simulink model "FKtest"  (Simulink 6.6)
settings: Solver=ode4  StartTime=0.0  StopTime=400  FixedStep=0.05  RelTol=1e-3
undefined symbols (not defined in the file or in its folder): amp2, vessel
libraries: marine_gnc x21, simulink x5
(part 2 of 3)

== system FKtest/Subsystem2/Subsystem ==
  In1 : Inport
  In2 : Inport  Port=2
  Integrator : Integrator
  Product4 : Product  Inputs=*/  RndMeth=Zero
  Out1 : Outport
  wires:
  Integrator/1 -> Product4/1
  In1/1 -> Integrator/1
  Product4/1 -> Out1/1
  In2/1 -> Product4/2

== system FKtest/Subsystem2/Subsystem1 ==
  In1 : Inport
  In2 : Inport  Port=2
  Integrator : Integrator
  Product4 : Product  Inputs=*/  RndMeth=Zero
  Out1 : Outport
  wires:
  Integrator/1 -> Product4/1
  In1/1 -> Integrator/1
  Product4/1 -> Out1/1
  In2/1 -> Product4/2

== system FKtest/Subsystem3/Subsystem ==
  In1 : Inport
  In2 : Inport  Port=2
  Integrator : Integrator
  Product4 : Product  Inputs=*/  RndMeth=Zero
  Out1 : Outport
  wires:
  Integrator/1 -> Product4/1
  In1/1 -> Integrator/1
  Product4/1 -> Out1/1
  In2/1 -> Product4/2

== system FKtest/Subsystem3/Subsystem1 ==
  In1 : Inport
  In2 : Inport  Port=2
  Integrator : Integrator
  Product4 : Product  Inputs=*/  RndMeth=Zero
  Out1 : Outport
  wires:
  Integrator/1 -> Product4/1
  In1/1 -> Integrator/1
  Product4/1 -> Out1/1
  In2/1 -> Product4/2

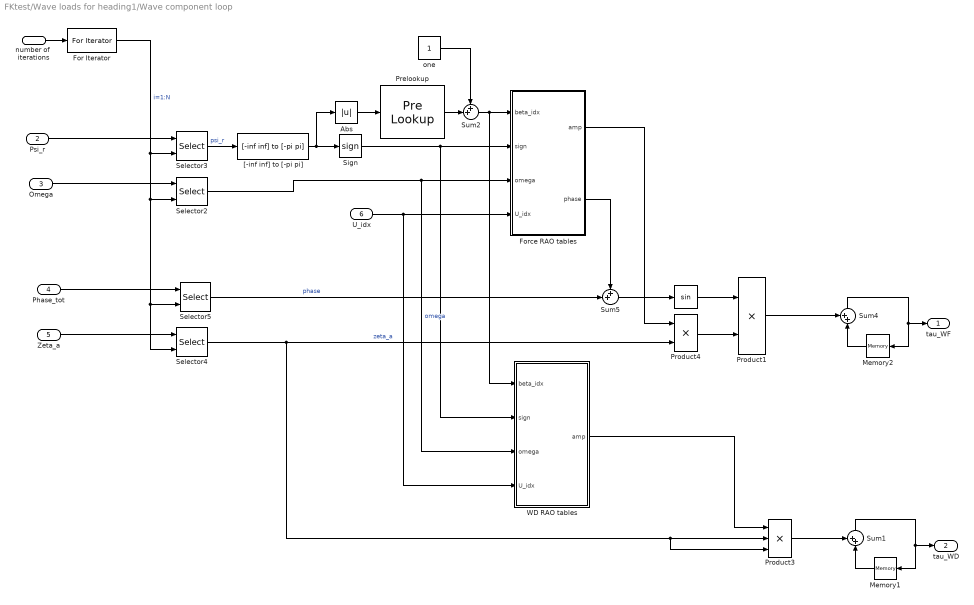
== system FKtest/Wave loads for heading1/Wave component loop ==
  number of  iterations : Inport
  Psi_r : Inport  Port=2
  Omega : Inport  Port=3
  Phase_tot : Inport  Port=4
  Zeta_a : Inport  Port=5
  U_idx : Inport  Port=6
  "                " : Trigonometry
  Abs : Abs  SaturateOnIntegerOverflow=on
  For Iterator : ForIterator  ResetStates=reset  IterationSource=external  IterationVariableDataType=double
  Force RAO tables : Subsystem  AncestorBlock=marine_gnc/Models/Environmental Loads/Utilities/RAO tables  mask(RAO table lookup){RAO_Freq=ForceRAO_Freq, RAO_Dir=RAO_Dir, RAO_Vel=RAO_Vel, RAO_Amp=ForceRAO_Amp, RAO_Phase=ForceRAO_Phase}
      mask prompts: RAO_Freq "Vector of frequencies (rad/s)"; RAO_Dir "Vector of directions (rad)"; RAO_Vel "Vector of velocities (m/s)"; RAO_Amp "6DOF Cell array with tables of Amplitudes"; RAO_Phase "6DOF Cell array with tables of Phases (rad)"
      mask help:
      | Perform 3D table lookup in 6DOF RAO amplitudes and phases, using the relative wave heading psi_r, wave frequency omega and vessel velocity vel as inputs. See documentation of the Motion RAO block or Force RAO block for details. A warning is issued if the input is outside the range spanned by the RAOs.
      |
      | Copyright (C) NTNU 2005
      |
      | Author: Oyvind N. Smogeli, 2005-05-03
  Memory1 : Memory  Orientation=left  X0=[0 0 0 0 0 0]'  InheritSampleTime=on
  Memory2 : Memory  Orientation=left  X0=[0 0 0 0 0 0]'  InheritSampleTime=on
  Prelookup : PreLookup  BreakpointsData=vessel.headings  BeginIndexSearchUsingPreviousIndexResult=on  OutputOnlyTheIndex=on
  Product1 : Product  SaturateOnIntegerOverflow=on
  Product3 : Product  Inputs=3  SaturateOnIntegerOverflow=on
  Product4 : Product  SaturateOnIntegerOverflow=on
  Selector{2..5} (4 alike) : Selector  IndexOptions=Index vector (port)  Indices=[1 3]  OutputSizes=1
  Sign : Signum
  Sum1 : Sum  Orientation=up  Inputs=++|  SaturateOnIntegerOverflow=on
  Sum2 : Sum  Inputs=++|
  Sum4 : Sum  Orientation=up  Inputs=++|  SaturateOnIntegerOverflow=on
  Sum5 : Sum  Inputs=++|  SaturateOnIntegerOverflow=on
  WD RAO tables : Subsystem  AncestorBlock=marine_gnc/Models/Environmental Loads/Utilities/RAO tables  mask(RAO table lookup){RAO_Freq=ForceRAO_Freq, RAO_Dir=RAO_Dir, RAO_Vel=RAO_Vel, RAO_Amp=ForceRAO_Amp, RAO_Phase=ForceRAO_Phase}
      mask prompts: RAO_Freq "Vector of frequencies (rad/s)"; RAO_Dir "Vector of directions (rad)"; RAO_Vel "Vector of velocities (m/s)"; RAO_Amp "6DOF Cell array with tables of Amplitudes"; RAO_Phase "6DOF Cell array with tables of Phases (rad)"
      mask help:
      | Perform 3D table lookup in 6DOF RAO amplitudes and phases, using the relative wave heading psi_r, wave frequency omega and vessel velocity vel as inputs. See documentation of the Motion RAO block or Force RAO block for details. A warning is issued if the input is outside the range spanned by the RAOs.
      |
      | Copyright (C) NTNU 2005
      |
      | Author: Oyvind N. Smogeli, 2005-05-03
  "[-inf inf] to [-pi pi]" : marine_gnc/Utilities/Math Operations/[-inf inf] to [-pi pi]  SystemSampleTime=-1
  one : Constant
  tau_WF : Outport
  tau_WD : Outport  Port=2
  wires:
  Selector4/1 -> Product4/2, Product3/2, Product3/3  "zeta_a"
  Sum5/1 -> "                "/1
  Zeta_a/1 -> Selector4/1
  Phase_tot/1 -> Selector5/1
  Force RAO tables/2(phase) -> Sum5/1
  Force RAO tables/1(amp) -> Product4/1
  U_idx/1 -> Force RAO tables/4(U_idx), WD RAO tables/4(U_idx)
  Psi_r/1 -> Selector3/1
  For Iterator/1 -> Selector3/2, Selector2/2, Selector5/2, Selector4/2  "i=1:N"
  Omega/1 -> Selector2/1
  number of  iterations/1 -> For Iterator/1
  Sum4/1 -> Memory2/1, tau_WF/1
  Memory2/1 -> Sum4/2
  Product1/1 -> Sum4/1
  Selector5/1 -> Sum5/2  "phase"
  Selector2/1 -> Force RAO tables/3(omega), WD RAO tables/3(omega)  "omega"
  Selector3/1 -> "[-inf inf] to [-pi pi]"/1  "psi_r"
  "                "/1 -> Product1/1
  Product4/1 -> Product1/2
  one/1 -> Sum2/1
  Sum2/1 -> Force RAO tables/1(beta_idx), WD RAO tables/1(beta_idx)
  Prelookup/1 -> Sum2/2
  Abs/1 -> Prelookup/1
  Sign/1 -> Force RAO tables/2(sign), WD RAO tables/2(sign)
  Sum1/1 -> Memory1/1, tau_WD/1
  Memory1/1 -> Sum1/2
  Product3/1 -> Sum1/1
  WD RAO tables/1(amp) -> Product3/1
  "[-inf inf] to [-pi pi]"/1 -> Abs/1, Sign/1

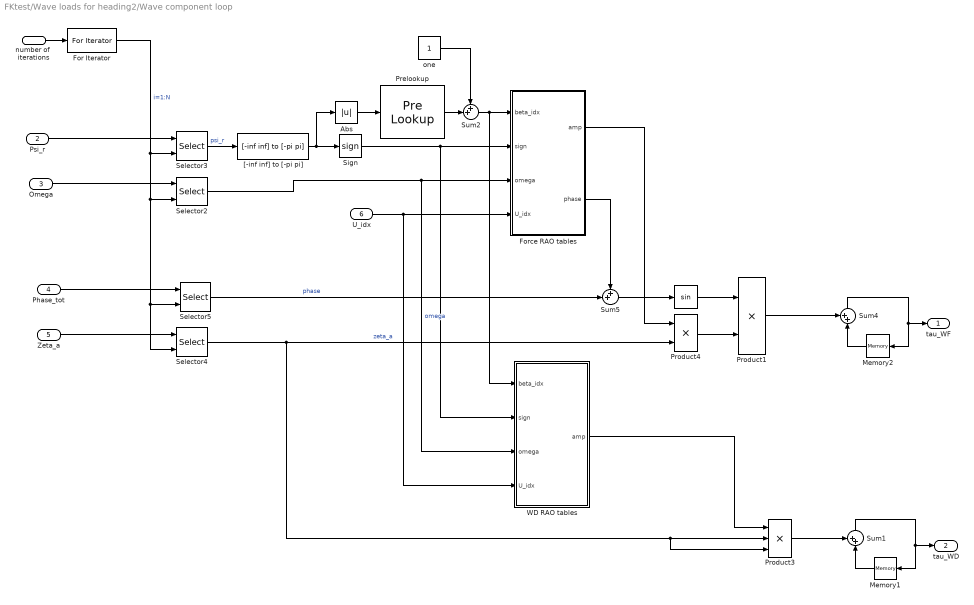
== system FKtest/Wave loads for heading2/Wave component loop ==
  number of  iterations : Inport
  Psi_r : Inport  Port=2
  Omega : Inport  Port=3
  Phase_tot : Inport  Port=4
  Zeta_a : Inport  Port=5
  U_idx : Inport  Port=6
  "                " : Trigonometry
  Abs : Abs  SaturateOnIntegerOverflow=on
  For Iterator : ForIterator  ResetStates=reset  IterationSource=external  IterationVariableDataType=double
  Force RAO tables : Subsystem  AncestorBlock=marine_gnc/Models/Environmental Loads/Utilities/RAO tables  mask(RAO table lookup){RAO_Freq=ForceRAO_Freq, RAO_Dir=RAO_Dir, RAO_Vel=RAO_Vel, RAO_Amp=ForceRAO_Amp, RAO_Phase=ForceRAO_Phase}
      mask prompts: RAO_Freq "Vector of frequencies (rad/s)"; RAO_Dir "Vector of directions (rad)"; RAO_Vel "Vector of velocities (m/s)"; RAO_Amp "6DOF Cell array with tables of Amplitudes"; RAO_Phase "6DOF Cell array with tables of Phases (rad)"
      mask help:
      | Perform 3D table lookup in 6DOF RAO amplitudes and phases, using the relative wave heading psi_r, wave frequency omega and vessel velocity vel as inputs. See documentation of the Motion RAO block or Force RAO block for details. A warning is issued if the input is outside the range spanned by the RAOs.
      |
      | Copyright (C) NTNU 2005
      |
      | Author: Oyvind N. Smogeli, 2005-05-03
  Memory1 : Memory  Orientation=left  X0=[0 0 0 0 0 0]'  InheritSampleTime=on
  Memory2 : Memory  Orientation=left  X0=[0 0 0 0 0 0]'  InheritSampleTime=on
  Prelookup : PreLookup  BreakpointsData=vessel.headings  BeginIndexSearchUsingPreviousIndexResult=on  OutputOnlyTheIndex=on
  Product1 : Product  SaturateOnIntegerOverflow=on
  Product3 : Product  Inputs=3  SaturateOnIntegerOverflow=on
  Product4 : Product  SaturateOnIntegerOverflow=on
  Selector{2..5} (4 alike) : Selector  IndexOptions=Index vector (port)  Indices=[1 3]  OutputSizes=1
  Sign : Signum
  Sum1 : Sum  Orientation=up  Inputs=++|  SaturateOnIntegerOverflow=on
  Sum2 : Sum  Inputs=++|
  Sum4 : Sum  Orientation=up  Inputs=++|  SaturateOnIntegerOverflow=on
  Sum5 : Sum  Inputs=++|  SaturateOnIntegerOverflow=on
  WD RAO tables : Subsystem  AncestorBlock=marine_gnc/Models/Environmental Loads/Utilities/RAO tables  mask(RAO table lookup){RAO_Freq=ForceRAO_Freq, RAO_Dir=RAO_Dir, RAO_Vel=RAO_Vel, RAO_Amp=ForceRAO_Amp, RAO_Phase=ForceRAO_Phase}
      mask prompts: RAO_Freq "Vector of frequencies (rad/s)"; RAO_Dir "Vector of directions (rad)"; RAO_Vel "Vector of velocities (m/s)"; RAO_Amp "6DOF Cell array with tables of Amplitudes"; RAO_Phase "6DOF Cell array with tables of Phases (rad)"
      mask help:
      | Perform 3D table lookup in 6DOF RAO amplitudes and phases, using the relative wave heading psi_r, wave frequency omega and vessel velocity vel as inputs. See documentation of the Motion RAO block or Force RAO block for details. A warning is issued if the input is outside the range spanned by the RAOs.
      |
      | Copyright (C) NTNU 2005
      |
      | Author: Oyvind N. Smogeli, 2005-05-03
  "[-inf inf] to [-pi pi]" : marine_gnc/Utilities/Math Operations/[-inf inf] to [-pi pi]  SystemSampleTime=-1
  one : Constant
  tau_WF : Outport
  tau_WD : Outport  Port=2
  wires:
  Selector4/1 -> Product4/2, Product3/2, Product3/3  "zeta_a"
  Sum5/1 -> "                "/1
  Zeta_a/1 -> Selector4/1
  Phase_tot/1 -> Selector5/1
  Force RAO tables/2(phase) -> Sum5/1
  Force RAO tables/1(amp) -> Product4/1
  U_idx/1 -> Force RAO tables/4(U_idx), WD RAO tables/4(U_idx)
  Psi_r/1 -> Selector3/1
  For Iterator/1 -> Selector3/2, Selector2/2, Selector5/2, Selector4/2  "i=1:N"
  Omega/1 -> Selector2/1
  number of  iterations/1 -> For Iterator/1
  Sum4/1 -> Memory2/1, tau_WF/1
  Memory2/1 -> Sum4/2
  Product1/1 -> Sum4/1
  Selector5/1 -> Sum5/2  "phase"
  Selector2/1 -> Force RAO tables/3(omega), WD RAO tables/3(omega)  "omega"
  Selector3/1 -> "[-inf inf] to [-pi pi]"/1  "psi_r"
  "                "/1 -> Product1/1
  Product4/1 -> Product1/2
  one/1 -> Sum2/1
  Sum2/1 -> Force RAO tables/1(beta_idx), WD RAO tables/1(beta_idx)
  Prelookup/1 -> Sum2/2
  Abs/1 -> Prelookup/1
  Sign/1 -> Force RAO tables/2(sign), WD RAO tables/2(sign)
  Sum1/1 -> Memory1/1, tau_WD/1
  Memory1/1 -> Sum1/2
  Product3/1 -> Sum1/1
  WD RAO tables/1(amp) -> Product3/1
  "[-inf inf] to [-pi pi]"/1 -> Abs/1, Sign/1

== system FKtest/3 DOF wave drift/Wave component loop/WD tables ==
  psi_r : Inport
  omega : Inport  Port=2
  vel : Inport  Port=3
  Abs : Abs  SaturateOnIntegerOverflow=on
  Amplitude table lookup1 : simulink/Lookup Tables/Lookup Table (n-D)  numDimsPopupSelect=3  bp1=RAO_Freq  bp2=RAO_Dir  bp3=RAO_Vel  bp4=[1:3]  bpcell={ [1:3], [1:3] }  explicitNumDims=2  searchMode=Binary Search  cacheBpFlag=off  vectorInputFlag=off  tableData=RAO_Amp{1}  interpMethod=None - Flat  extrapMethod=Linear  rangeErrorMode=Warning
  Amplitude table lookup2 : simulink/Lookup Tables/Lookup Table (n-D)  numDimsPopupSelect=3  bp1=RAO_Freq  bp2=RAO_Dir  bp3=RAO_Vel  bp4=[1:3]  bpcell={ [1:3], [1:3] }  explicitNumDims=2  searchMode=Binary Search  cacheBpFlag=off  vectorInputFlag=off  tableData=RAO_Amp{2}  interpMethod=None - Flat  extrapMethod=Linear  rangeErrorMode=None
  Amplitude table lookup6 : simulink/Lookup Tables/Lookup Table (n-D)  numDimsPopupSelect=3  bp1=RAO_Freq  bp2=RAO_Dir  bp3=RAO_Vel  bp4=[1:3]  bpcell={ [1:3], [1:3] }  explicitNumDims=2  searchMode=Binary Search  cacheBpFlag=off  vectorInputFlag=off  tableData=RAO_Amp{3}  interpMethod=None - Flat  extrapMethod=Linear  rangeErrorMode=None
  Constant : Constant  Value=0
  Mux1 : Mux  Inputs=6
  Product1 : Product  Inputs=**  SaturateOnIntegerOverflow=on
  Product3 : Product  Inputs=**  SaturateOnIntegerOverflow=on
  Sign : Signum
  "[-inf inf] to [-pi pi]" : marine_gnc/Utilities/Math Operations/[-inf inf] to [-pi pi]  SystemSampleTime=-1
  amp : Outport
  wires:
  Mux1/1 -> amp/1
  vel/1 -> Amplitude table lookup2/3, Amplitude table lookup6/3, Amplitude table lookup1/3
  psi_r/1 -> "[-inf inf] to [-pi pi]"/1
  Amplitude table lookup6/1 -> Product3/2
  Product3/1 -> Mux1/6
  Constant/1 -> Mux1/4, Mux1/3, Mux1/5
  Sign/1 -> Product1/1, Product3/1
  Amplitude table lookup2/1 -> Product1/2
  Product1/1 -> Mux1/2
  Abs/1 -> Amplitude table lookup2/2, Amplitude table lookup6/2, Amplitude table lookup1/2
  "[-inf inf] to [-pi pi]"/1 -> Sign/1, Abs/1
  omega/1 -> Amplitude table lookup2/1, Amplitude table lookup6/1, Amplitude table lookup1/1
  Amplitude table lookup1/1 -> Mux1/1

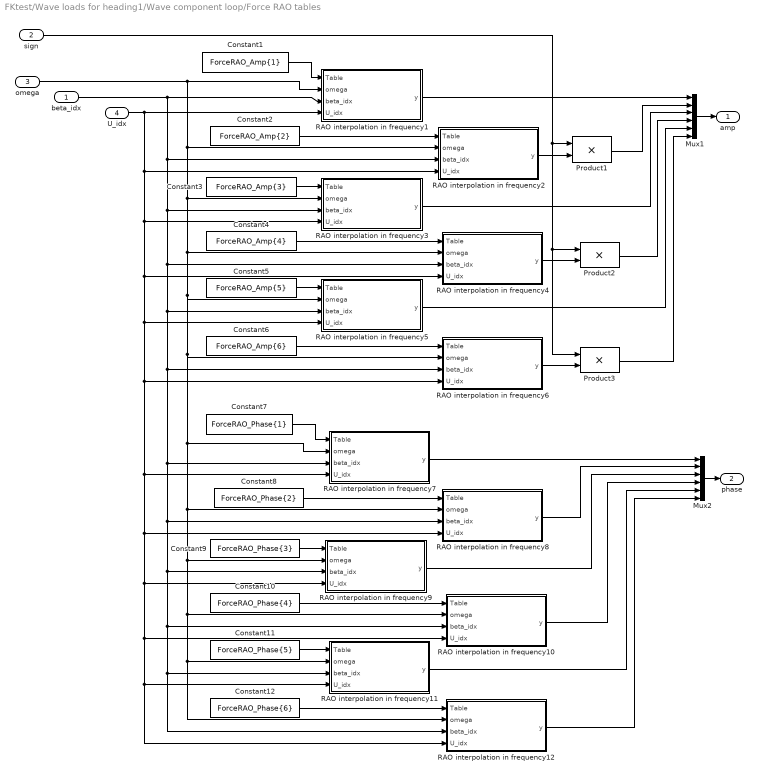
== system FKtest/Wave loads for heading1/Wave component loop/Force RAO tables ==
  beta_idx : Inport
  sign : Inport  Port=2
  omega : Inport  Port=3
  U_idx : Inport  Port=4
  Constant1 : Constant  Value=ForceRAO_Amp{1}
  Constant10 : Constant  Value=ForceRAO_Phase{4}
  Constant11 : Constant  Value=ForceRAO_Phase{5}
  Constant12 : Constant  Value=ForceRAO_Phase{6}
  Constant2 : Constant  Value=ForceRAO_Amp{2}
  Constant3 : Constant  Value=ForceRAO_Amp{3}
  Constant4 : Constant  Value=ForceRAO_Amp{4}
  Constant5 : Constant  Value=ForceRAO_Amp{5}
  Constant6 : Constant  Value=ForceRAO_Amp{6}
  Constant7 : Constant  Value=ForceRAO_Phase{1}
  Constant8 : Constant  Value=ForceRAO_Phase{2}
  Constant9 : Constant  Value=ForceRAO_Phase{3}
  Mux1 : Mux  Inputs=6
  Mux2 : Mux  Inputs=6
  Product1 : Product  Inputs=**  SaturateOnIntegerOverflow=on
  Product2 : Product  Inputs=**  SaturateOnIntegerOverflow=on
  Product3 : Product  Inputs=**  SaturateOnIntegerOverflow=on
  RAO interpolation in frequency1 : Subsystem
  RAO interpolation in frequency10 : Subsystem
  RAO interpolation in frequency11 : Subsystem
  RAO interpolation in frequency12 : Subsystem
  RAO interpolation in frequency2 : Subsystem
  RAO interpolation in frequency3 : Subsystem
  RAO interpolation in frequency4 : Subsystem
  RAO interpolation in frequency5 : Subsystem
  RAO interpolation in frequency6 : Subsystem
  RAO interpolation in frequency7 : Subsystem
  RAO interpolation in frequency8 : Subsystem
  RAO interpolation in frequency9 : Subsystem
  amp : Outport
  phase : Outport  Port=2
  wires:
  Mux1/1 -> amp/1
  Mux2/1 -> phase/1
  sign/1 -> Product3/1, Product2/1, Product1/1
  RAO interpolation in frequency6/1(y) -> Product3/2
  Product3/1 -> Mux1/6
  Product2/1 -> Mux1/4
  RAO interpolation in frequency2/1(y) -> Product1/2
  Product1/1 -> Mux1/2
  RAO interpolation in frequency5/1(y) -> Mux1/5
  RAO interpolation in frequency3/1(y) -> Mux1/3
  omega/1 -> RAO interpolation in frequency1/2(omega), RAO interpolation in frequency11/2(omega), RAO interpolation in frequency12/2(omega), RAO interpolation in frequency10/2(omega), RAO interpolation in frequency9/2(omega), RAO interpolation in frequency8/2(omega), RAO interpolation in frequency7/2(omega), RAO interpolation in frequency6/2(omega), RAO interpolation in frequency5/2(omega), RAO interpolation in frequency4/2(omega), RAO interpolation in frequency3/2(omega), RAO interpolation in frequency2/2(omega)
  RAO interpolation in frequency1/1(y) -> Mux1/1
  Constant1/1 -> RAO interpolation in frequency1/1(Table)
  Constant2/1 -> RAO interpolation in frequency2/1(Table)
  Constant3/1 -> RAO interpolation in frequency3/1(Table)
  U_idx/1 -> RAO interpolation in frequency1/4(U_idx), RAO interpolation in frequency11/4(U_idx), RAO interpolation in frequency12/4(U_idx), RAO interpolation in frequency10/4(U_idx), RAO interpolation in frequency9/4(U_idx), RAO interpolation in frequency8/4(U_idx), RAO interpolation in frequency7/4(U_idx), RAO interpolation in frequency6/4(U_idx), RAO interpolation in frequency5/4(U_idx), RAO interpolation in frequency4/4(U_idx), RAO interpolation in frequency3/4(U_idx), RAO interpolation in frequency2/4(U_idx)
  Constant4/1 -> RAO interpolation in frequency4/1(Table)
  RAO interpolation in frequency4/1(y) -> Product2/2
  Constant5/1 -> RAO interpolation in frequency5/1(Table)
  Constant6/1 -> RAO interpolation in frequency6/1(Table)
  RAO interpolation in frequency12/1(y) -> Mux2/6
  RAO interpolation in frequency8/1(y) -> Mux2/2
  Constant7/1 -> RAO interpolation in frequency7/1(Table)
  Constant8/1 -> RAO interpolation in frequency8/1(Table)
  Constant9/1 -> RAO interpolation in frequency9/1(Table)
  Constant10/1 -> RAO interpolation in frequency10/1(Table)
  RAO interpolation in frequency10/1(y) -> Mux2/4
  Constant11/1 -> RAO interpolation in frequency11/1(Table)
  Constant12/1 -> RAO interpolation in frequency12/1(Table)
  beta_idx/1 -> RAO interpolation in frequency11/3(beta_idx), RAO interpolation in frequency12/3(beta_idx), RAO interpolation in frequency10/3(beta_idx), RAO interpolation in frequency9/3(beta_idx), RAO interpolation in frequency8/3(beta_idx), RAO interpolation in frequency7/3(beta_idx), RAO interpolation in frequency6/3(beta_idx), RAO interpolation in frequency5/3(beta_idx), RAO interpolation in frequency4/3(beta_idx), RAO interpolation in frequency3/3(beta_idx), RAO interpolation in frequency2/3(beta_idx), RAO interpolation in frequency1/3(beta_idx)
  RAO interpolation in frequency7/1(y) -> Mux2/1
  RAO interpolation in frequency9/1(y) -> Mux2/3
  RAO interpolation in frequency11/1(y) -> Mux2/5

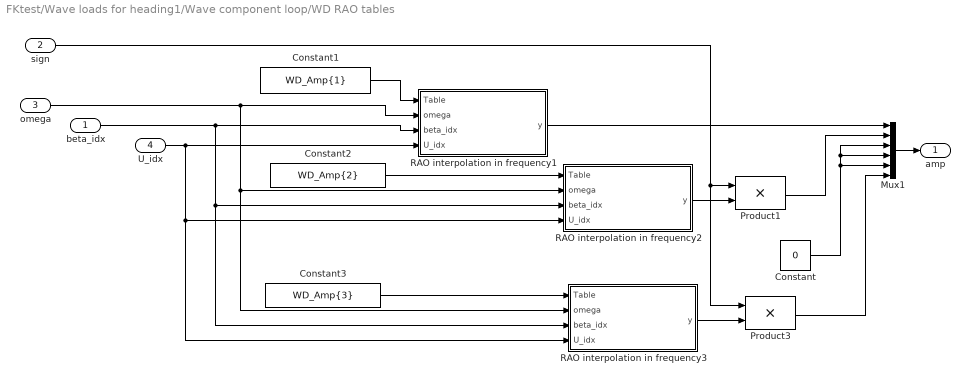
== system FKtest/Wave loads for heading1/Wave component loop/WD RAO tables ==
  beta_idx : Inport
  sign : Inport  Port=2
  omega : Inport  Port=3
  U_idx : Inport  Port=4
  Constant : Constant  Value=0
  Constant1 : Constant  Value=WD_Amp{1}
  Constant2 : Constant  Value=WD_Amp{2}
  Constant3 : Constant  Value=WD_Amp{3}
  Mux1 : Mux  Inputs=6
  Product1 : Product  Inputs=**  SaturateOnIntegerOverflow=on
  Product3 : Product  Inputs=**  SaturateOnIntegerOverflow=on
  RAO interpolation in frequency1 : Subsystem
  RAO interpolation in frequency2 : Subsystem
  RAO interpolation in frequency3 : Subsystem
  amp : Outport
  wires:
  Mux1/1 -> amp/1
  sign/1 -> Product1/1, Product3/1
  RAO interpolation in frequency3/1(y) -> Product3/2
  Product3/1 -> Mux1/6
  RAO interpolation in frequency2/1(y) -> Product1/2
  Product1/1 -> Mux1/2
  omega/1 -> RAO interpolation in frequency2/2(omega), RAO interpolation in frequency3/2(omega), RAO interpolation in frequency1/2(omega)
  RAO interpolation in frequency1/1(y) -> Mux1/1
  Constant1/1 -> RAO interpolation in frequency1/1(Table)
  Constant2/1 -> RAO interpolation in frequency2/1(Table)
  U_idx/1 -> RAO interpolation in frequency2/4(U_idx), RAO interpolation in frequency3/4(U_idx), RAO interpolation in frequency1/4(U_idx)
  Constant3/1 -> RAO interpolation in frequency3/1(Table)
  beta_idx/1 -> RAO interpolation in frequency2/3(beta_idx), RAO interpolation in frequency3/3(beta_idx), RAO interpolation in frequency1/3(beta_idx)
  Constant/1 -> Mux1/3, Mux1/4, Mux1/5

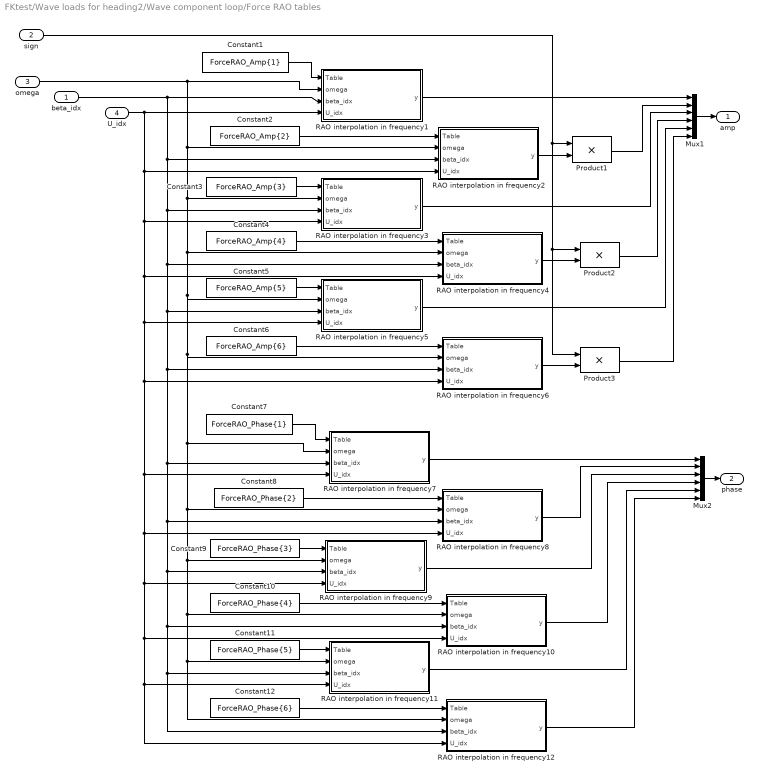
== system FKtest/Wave loads for heading2/Wave component loop/Force RAO tables ==
  beta_idx : Inport
  sign : Inport  Port=2
  omega : Inport  Port=3
  U_idx : Inport  Port=4
  Constant1 : Constant  Value=ForceRAO_Amp{1}
  Constant10 : Constant  Value=ForceRAO_Phase{4}
  Constant11 : Constant  Value=ForceRAO_Phase{5}
  Constant12 : Constant  Value=ForceRAO_Phase{6}
  Constant2 : Constant  Value=ForceRAO_Amp{2}
  Constant3 : Constant  Value=ForceRAO_Amp{3}
  Constant4 : Constant  Value=ForceRAO_Amp{4}
  Constant5 : Constant  Value=ForceRAO_Amp{5}
  Constant6 : Constant  Value=ForceRAO_Amp{6}
  Constant7 : Constant  Value=ForceRAO_Phase{1}
  Constant8 : Constant  Value=ForceRAO_Phase{2}
  Constant9 : Constant  Value=ForceRAO_Phase{3}
  Mux1 : Mux  Inputs=6
  Mux2 : Mux  Inputs=6
  Product1 : Product  Inputs=**  SaturateOnIntegerOverflow=on
  Product2 : Product  Inputs=**  SaturateOnIntegerOverflow=on
  Product3 : Product  Inputs=**  SaturateOnIntegerOverflow=on
  RAO interpolation in frequency1 : Subsystem
  RAO interpolation in frequency10 : Subsystem
  RAO interpolation in frequency11 : Subsystem
  RAO interpolation in frequency12 : Subsystem
  RAO interpolation in frequency2 : Subsystem
  RAO interpolation in frequency3 : Subsystem
  RAO interpolation in frequency4 : Subsystem
  RAO interpolation in frequency5 : Subsystem
  RAO interpolation in frequency6 : Subsystem
  RAO interpolation in frequency7 : Subsystem
  RAO interpolation in frequency8 : Subsystem
  RAO interpolation in frequency9 : Subsystem
  amp : Outport
  phase : Outport  Port=2
  wires:
  Mux1/1 -> amp/1
  Mux2/1 -> phase/1
  sign/1 -> Product3/1, Product2/1, Product1/1
  RAO interpolation in frequency6/1(y) -> Product3/2
  Product3/1 -> Mux1/6
  Product2/1 -> Mux1/4
  RAO interpolation in frequency2/1(y) -> Product1/2
  Product1/1 -> Mux1/2
  RAO interpolation in frequency5/1(y) -> Mux1/5
  RAO interpolation in frequency3/1(y) -> Mux1/3
  omega/1 -> RAO interpolation in frequency1/2(omega), RAO interpolation in frequency11/2(omega), RAO interpolation in frequency12/2(omega), RAO interpolation in frequency10/2(omega), RAO interpolation in frequency9/2(omega), RAO interpolation in frequency8/2(omega), RAO interpolation in frequency7/2(omega), RAO interpolation in frequency6/2(omega), RAO interpolation in frequency5/2(omega), RAO interpolation in frequency4/2(omega), RAO interpolation in frequency3/2(omega), RAO interpolation in frequency2/2(omega)
  RAO interpolation in frequency1/1(y) -> Mux1/1
  Constant1/1 -> RAO interpolation in frequency1/1(Table)
  Constant2/1 -> RAO interpolation in frequency2/1(Table)
  Constant3/1 -> RAO interpolation in frequency3/1(Table)
  U_idx/1 -> RAO interpolation in frequency1/4(U_idx), RAO interpolation in frequency11/4(U_idx), RAO interpolation in frequency12/4(U_idx), RAO interpolation in frequency10/4(U_idx), RAO interpolation in frequency9/4(U_idx), RAO interpolation in frequency8/4(U_idx), RAO interpolation in frequency7/4(U_idx), RAO interpolation in frequency6/4(U_idx), RAO interpolation in frequency5/4(U_idx), RAO interpolation in frequency4/4(U_idx), RAO interpolation in frequency3/4(U_idx), RAO interpolation in frequency2/4(U_idx)
  Constant4/1 -> RAO interpolation in frequency4/1(Table)
  RAO interpolation in frequency4/1(y) -> Product2/2
  Constant5/1 -> RAO interpolation in frequency5/1(Table)
  Constant6/1 -> RAO interpolation in frequency6/1(Table)
  RAO interpolation in frequency12/1(y) -> Mux2/6
  RAO interpolation in frequency8/1(y) -> Mux2/2
  Constant7/1 -> RAO interpolation in frequency7/1(Table)
  Constant8/1 -> RAO interpolation in frequency8/1(Table)
  Constant9/1 -> RAO interpolation in frequency9/1(Table)
  Constant10/1 -> RAO interpolation in frequency10/1(Table)
  RAO interpolation in frequency10/1(y) -> Mux2/4
  Constant11/1 -> RAO interpolation in frequency11/1(Table)
  Constant12/1 -> RAO interpolation in frequency12/1(Table)
  beta_idx/1 -> RAO interpolation in frequency11/3(beta_idx), RAO interpolation in frequency12/3(beta_idx), RAO interpolation in frequency10/3(beta_idx), RAO interpolation in frequency9/3(beta_idx), RAO interpolation in frequency8/3(beta_idx), RAO interpolation in frequency7/3(beta_idx), RAO interpolation in frequency6/3(beta_idx), RAO interpolation in frequency5/3(beta_idx), RAO interpolation in frequency4/3(beta_idx), RAO interpolation in frequency3/3(beta_idx), RAO interpolation in frequency2/3(beta_idx), RAO interpolation in frequency1/3(beta_idx)
  RAO interpolation in frequency7/1(y) -> Mux2/1
  RAO interpolation in frequency9/1(y) -> Mux2/3
  RAO interpolation in frequency11/1(y) -> Mux2/5

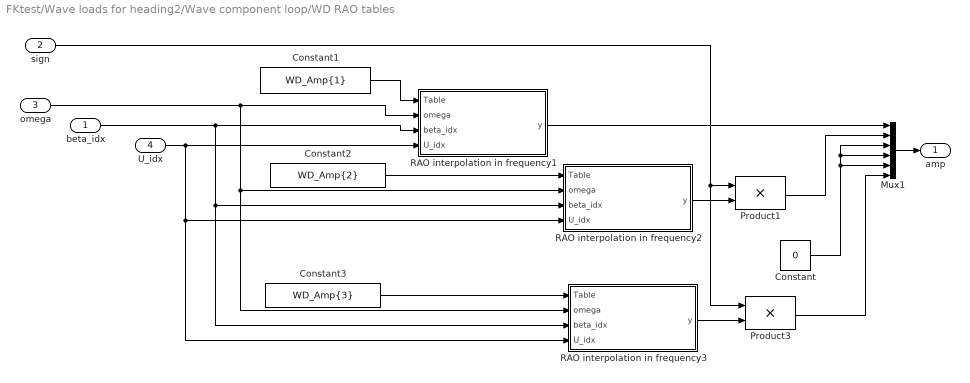
== system FKtest/Wave loads for heading2/Wave component loop/WD RAO tables ==
  beta_idx : Inport
  sign : Inport  Port=2
  omega : Inport  Port=3
  U_idx : Inport  Port=4
  Constant : Constant  Value=0
  Constant1 : Constant  Value=WD_Amp{1}
  Constant2 : Constant  Value=WD_Amp{2}
  Constant3 : Constant  Value=WD_Amp{3}
  Mux1 : Mux  Inputs=6
  Product1 : Product  Inputs=**  SaturateOnIntegerOverflow=on
  Product3 : Product  Inputs=**  SaturateOnIntegerOverflow=on
  RAO interpolation in frequency1 : Subsystem
  RAO interpolation in frequency2 : Subsystem
  RAO interpolation in frequency3 : Subsystem
  amp : Outport
  wires:
  Mux1/1 -> amp/1
  sign/1 -> Product1/1, Product3/1
  RAO interpolation in frequency3/1(y) -> Product3/2
  Product3/1 -> Mux1/6
  RAO interpolation in frequency2/1(y) -> Product1/2
  Product1/1 -> Mux1/2
  omega/1 -> RAO interpolation in frequency2/2(omega), RAO interpolation in frequency3/2(omega), RAO interpolation in frequency1/2(omega)
  RAO interpolation in frequency1/1(y) -> Mux1/1
  Constant1/1 -> RAO interpolation in frequency1/1(Table)
  Constant2/1 -> RAO interpolation in frequency2/1(Table)
  U_idx/1 -> RAO interpolation in frequency2/4(U_idx), RAO interpolation in frequency3/4(U_idx), RAO interpolation in frequency1/4(U_idx)
  Constant3/1 -> RAO interpolation in frequency3/1(Table)
  beta_idx/1 -> RAO interpolation in frequency2/3(beta_idx), RAO interpolation in frequency3/3(beta_idx), RAO interpolation in frequency1/3(beta_idx)
  Constant/1 -> Mux1/3, Mux1/4, Mux1/5

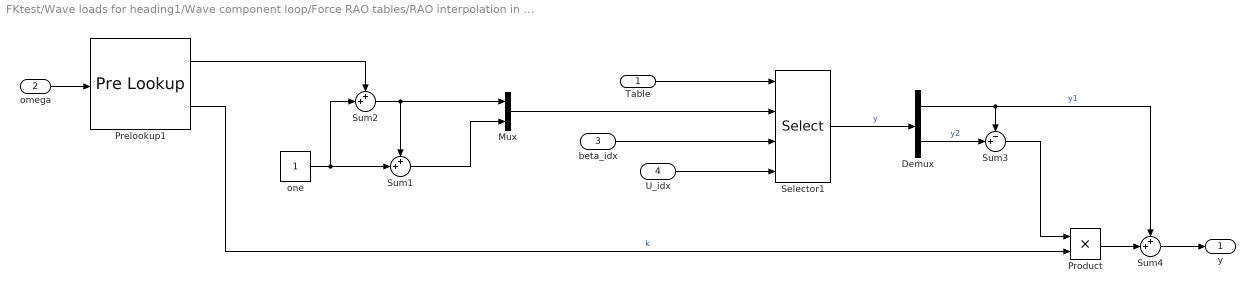
== system FKtest/Wave loads for heading1/Wave component loop/Force RAO tables/RAO interpolation in frequency1 ==
  Table : Inport
  omega : Inport  Port=2
  beta_idx : Inport  Port=3
  U_idx : Inport  Port=4
  Demux : Demux  Outputs=2
  Mux : Mux  Inputs=2
  Prelookup1 : PreLookup  BreakpointsData=vessel.forceRAO.w  BeginIndexSearchUsingPreviousIndexResult=on  ProcessOutOfRangeInput=Linear extrapolation
  Product : Product  RndMeth=Zero
  Selector1 : Selector  NumberOfDimensions=3  IndexOptions=Index vector (port),Index vector (port),Index vector (port)  Indices=[1 3],1,1  OutputSizes=1,1,1
  Sum1 : Sum  Inputs=++|
  Sum2 : Sum  Inputs=++|
  Sum3 : Sum  Inputs=-+|
  Sum4 : Sum  Inputs=++|
  one : Constant
  y : Outport
  wires:
  Prelookup1/1 -> Sum2/1
  Table/1 -> Selector1/1
  beta_idx/1 -> Selector1/3
  omega/1 -> Prelookup1/1
  U_idx/1 -> Selector1/4
  Sum4/1 -> y/1
  Sum3/1 -> Product/1
  Product/1 -> Sum4/2
  Demux/1 -> Sum4/1, Sum3/1  "y1"
  Demux/2 -> Sum3/2  "y2"
  Prelookup1/2 -> Product/2  "k"
  Selector1/1 -> Demux/1  "y"
  one/1 -> Sum1/2, Sum2/2
  Sum1/1 -> Mux/2
  Sum2/1 -> Sum1/1, Mux/1
  Mux/1 -> Selector1/2

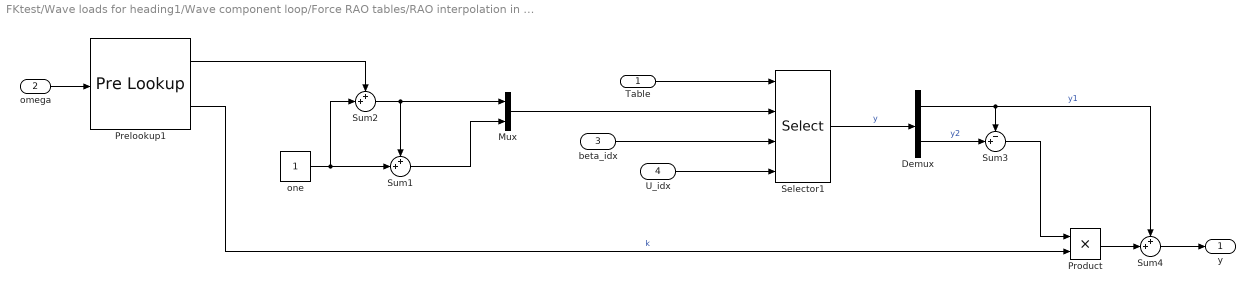
== system FKtest/Wave loads for heading1/Wave component loop/Force RAO tables/RAO interpolation in frequency10 ==
  Table : Inport
  omega : Inport  Port=2
  beta_idx : Inport  Port=3
  U_idx : Inport  Port=4
  Demux : Demux  Outputs=2
  Mux : Mux  Inputs=2
  Prelookup1 : PreLookup  BreakpointsData=vessel.forceRAO.w  BeginIndexSearchUsingPreviousIndexResult=on  ProcessOutOfRangeInput=Linear extrapolation
  Product : Product  RndMeth=Zero
  Selector1 : Selector  NumberOfDimensions=3  IndexOptions=Index vector (port),Index vector (port),Index vector (port)  Indices=[1 3],1,1  OutputSizes=1,1,1
  Sum1 : Sum  Inputs=++|
  Sum2 : Sum  Inputs=++|
  Sum3 : Sum  Inputs=-+|
  Sum4 : Sum  Inputs=++|
  one : Constant
  y : Outport
  wires:
  Prelookup1/1 -> Sum2/1
  Table/1 -> Selector1/1
  beta_idx/1 -> Selector1/3
  omega/1 -> Prelookup1/1
  U_idx/1 -> Selector1/4
  Sum4/1 -> y/1
  Sum3/1 -> Product/1
  Product/1 -> Sum4/2
  Demux/1 -> Sum4/1, Sum3/1  "y1"
  Demux/2 -> Sum3/2  "y2"
  Prelookup1/2 -> Product/2  "k"
  Selector1/1 -> Demux/1  "y"
  one/1 -> Sum1/2, Sum2/2
  Sum1/1 -> Mux/2
  Sum2/1 -> Sum1/1, Mux/1
  Mux/1 -> Selector1/2

== system FKtest/Wave loads for heading1/Wave component loop/Force RAO tables/RAO interpolation in frequency11 ==
  Table : Inport
  omega : Inport  Port=2
  beta_idx : Inport  Port=3
  U_idx : Inport  Port=4
  Demux : Demux  Outputs=2
  Mux : Mux  Inputs=2
  Prelookup1 : PreLookup  BreakpointsData=vessel.forceRAO.w  BeginIndexSearchUsingPreviousIndexResult=on  ProcessOutOfRangeInput=Linear extrapolation
  Product : Product  RndMeth=Zero
  Selector1 : Selector  NumberOfDimensions=3  IndexOptions=Index vector (port),Index vector (port),Index vector (port)  Indices=[1 3],1,1  OutputSizes=1,1,1
  Sum1 : Sum  Inputs=++|
  Sum2 : Sum  Inputs=++|
  Sum3 : Sum  Inputs=-+|
  Sum4 : Sum  Inputs=++|
  one : Constant
  y : Outport
  wires:
  Prelookup1/1 -> Sum2/1
  Table/1 -> Selector1/1
  beta_idx/1 -> Selector1/3
  omega/1 -> Prelookup1/1
  U_idx/1 -> Selector1/4
  Sum4/1 -> y/1
  Sum3/1 -> Product/1
  Product/1 -> Sum4/2
  Demux/1 -> Sum4/1, Sum3/1  "y1"
  Demux/2 -> Sum3/2  "y2"
  Prelookup1/2 -> Product/2  "k"
  Selector1/1 -> Demux/1  "y"
  one/1 -> Sum1/2, Sum2/2
  Sum1/1 -> Mux/2
  Sum2/1 -> Sum1/1, Mux/1
  Mux/1 -> Selector1/2

== system FKtest/Wave loads for heading1/Wave component loop/Force RAO tables/RAO interpolation in frequency12 ==
  Table : Inport
  omega : Inport  Port=2
  beta_idx : Inport  Port=3
  U_idx : Inport  Port=4
  Demux : Demux  Outputs=2
  Mux : Mux  Inputs=2
  Prelookup1 : PreLookup  BreakpointsData=vessel.forceRAO.w  BeginIndexSearchUsingPreviousIndexResult=on  ProcessOutOfRangeInput=Linear extrapolation
  Product : Product  RndMeth=Zero
  Selector1 : Selector  NumberOfDimensions=3  IndexOptions=Index vector (port),Index vector (port),Index vector (port)  Indices=[1 3],1,1  OutputSizes=1,1,1
  Sum1 : Sum  Inputs=++|
  Sum2 : Sum  Inputs=++|
  Sum3 : Sum  Inputs=-+|
  Sum4 : Sum  Inputs=++|
  one : Constant
  y : Outport
  wires:
  Prelookup1/1 -> Sum2/1
  Table/1 -> Selector1/1
  beta_idx/1 -> Selector1/3
  omega/1 -> Prelookup1/1
  U_idx/1 -> Selector1/4
  Sum4/1 -> y/1
  Sum3/1 -> Product/1
  Product/1 -> Sum4/2
  Demux/1 -> Sum4/1, Sum3/1  "y1"
  Demux/2 -> Sum3/2  "y2"
  Prelookup1/2 -> Product/2  "k"
  Selector1/1 -> Demux/1  "y"
  one/1 -> Sum1/2, Sum2/2
  Sum1/1 -> Mux/2
  Sum2/1 -> Sum1/1, Mux/1
  Mux/1 -> Selector1/2

== system FKtest/Wave loads for heading1/Wave component loop/Force RAO tables/RAO interpolation in frequency2 ==
  Table : Inport
  omega : Inport  Port=2
  beta_idx : Inport  Port=3
  U_idx : Inport  Port=4
  Demux : Demux  Outputs=2
  Mux : Mux  Inputs=2
  Prelookup1 : PreLookup  BreakpointsData=vessel.forceRAO.w  BeginIndexSearchUsingPreviousIndexResult=on  ProcessOutOfRangeInput=Linear extrapolation
  Product : Product  RndMeth=Zero
  Selector1 : Selector  NumberOfDimensions=3  IndexOptions=Index vector (port),Index vector (port),Index vector (port)  Indices=[1 3],1,1  OutputSizes=1,1,1
  Sum1 : Sum  Inputs=++|
  Sum2 : Sum  Inputs=++|
  Sum3 : Sum  Inputs=-+|
  Sum4 : Sum  Inputs=++|
  one : Constant
  y : Outport
  wires:
  Prelookup1/1 -> Sum2/1
  Table/1 -> Selector1/1
  beta_idx/1 -> Selector1/3
  omega/1 -> Prelookup1/1
  U_idx/1 -> Selector1/4
  Sum4/1 -> y/1
  Sum3/1 -> Product/1
  Product/1 -> Sum4/2
  Demux/1 -> Sum4/1, Sum3/1  "y1"
  Demux/2 -> Sum3/2  "y2"
  Prelookup1/2 -> Product/2  "k"
  Selector1/1 -> Demux/1  "y"
  one/1 -> Sum1/2, Sum2/2
  Sum1/1 -> Mux/2
  Sum2/1 -> Sum1/1, Mux/1
  Mux/1 -> Selector1/2

== system FKtest/Wave loads for heading1/Wave component loop/Force RAO tables/RAO interpolation in frequency3 ==
  Table : Inport
  omega : Inport  Port=2
  beta_idx : Inport  Port=3
  U_idx : Inport  Port=4
  Demux : Demux  Outputs=2
  Mux : Mux  Inputs=2
  Prelookup1 : PreLookup  BreakpointsData=vessel.forceRAO.w  BeginIndexSearchUsingPreviousIndexResult=on  ProcessOutOfRangeInput=Linear extrapolation
  Product : Product  RndMeth=Zero
  Selector1 : Selector  NumberOfDimensions=3  IndexOptions=Index vector (port),Index vector (port),Index vector (port)  Indices=[1 3],1,1  OutputSizes=1,1,1
  Sum1 : Sum  Inputs=++|
  Sum2 : Sum  Inputs=++|
  Sum3 : Sum  Inputs=-+|
  Sum4 : Sum  Inputs=++|
  one : Constant
  y : Outport
  wires:
  Prelookup1/1 -> Sum2/1
  Table/1 -> Selector1/1
  beta_idx/1 -> Selector1/3
  omega/1 -> Prelookup1/1
  U_idx/1 -> Selector1/4
  Sum4/1 -> y/1
  Sum3/1 -> Product/1
  Product/1 -> Sum4/2
  Demux/1 -> Sum4/1, Sum3/1  "y1"
  Demux/2 -> Sum3/2  "y2"
  Prelookup1/2 -> Product/2  "k"
  Selector1/1 -> Demux/1  "y"
  one/1 -> Sum1/2, Sum2/2
  Sum1/1 -> Mux/2
  Sum2/1 -> Sum1/1, Mux/1
  Mux/1 -> Selector1/2

== system FKtest/Wave loads for heading1/Wave component loop/Force RAO tables/RAO interpolation in frequency4 ==
  Table : Inport
  omega : Inport  Port=2
  beta_idx : Inport  Port=3
  U_idx : Inport  Port=4
  Demux : Demux  Outputs=2
  Mux : Mux  Inputs=2
  Prelookup1 : PreLookup  BreakpointsData=vessel.forceRAO.w  BeginIndexSearchUsingPreviousIndexResult=on  ProcessOutOfRangeInput=Linear extrapolation
  Product : Product  RndMeth=Zero
  Selector1 : Selector  NumberOfDimensions=3  IndexOptions=Index vector (port),Index vector (port),Index vector (port)  Indices=[1 3],1,1  OutputSizes=1,1,1
  Sum1 : Sum  Inputs=++|
  Sum2 : Sum  Inputs=++|
  Sum3 : Sum  Inputs=-+|
  Sum4 : Sum  Inputs=++|
  one : Constant
  y : Outport
  wires:
  Prelookup1/1 -> Sum2/1
  Table/1 -> Selector1/1
  beta_idx/1 -> Selector1/3
  omega/1 -> Prelookup1/1
  U_idx/1 -> Selector1/4
  Sum4/1 -> y/1
  Sum3/1 -> Product/1
  Product/1 -> Sum4/2
  Demux/1 -> Sum4/1, Sum3/1  "y1"
  Demux/2 -> Sum3/2  "y2"
  Prelookup1/2 -> Product/2  "k"
  Selector1/1 -> Demux/1  "y"
  one/1 -> Sum1/2, Sum2/2
  Sum1/1 -> Mux/2
  Sum2/1 -> Sum1/1, Mux/1
  Mux/1 -> Selector1/2

== system FKtest/Wave loads for heading1/Wave component loop/Force RAO tables/RAO interpolation in frequency5 ==
  Table : Inport
  omega : Inport  Port=2
  beta_idx : Inport  Port=3
  U_idx : Inport  Port=4
  Demux : Demux  Outputs=2
  Mux : Mux  Inputs=2
  Prelookup1 : PreLookup  BreakpointsData=vessel.forceRAO.w  BeginIndexSearchUsingPreviousIndexResult=on  ProcessOutOfRangeInput=Linear extrapolation
  Product : Product  RndMeth=Zero
  Selector1 : Selector  NumberOfDimensions=3  IndexOptions=Index vector (port),Index vector (port),Index vector (port)  Indices=[1 3],1,1  OutputSizes=1,1,1
  Sum1 : Sum  Inputs=++|
  Sum2 : Sum  Inputs=++|
  Sum3 : Sum  Inputs=-+|
  Sum4 : Sum  Inputs=++|
  one : Constant
  y : Outport
  wires:
  Prelookup1/1 -> Sum2/1
  Table/1 -> Selector1/1
  beta_idx/1 -> Selector1/3
  omega/1 -> Prelookup1/1
  U_idx/1 -> Selector1/4
  Sum4/1 -> y/1
  Sum3/1 -> Product/1
  Product/1 -> Sum4/2
  Demux/1 -> Sum4/1, Sum3/1  "y1"
  Demux/2 -> Sum3/2  "y2"
  Prelookup1/2 -> Product/2  "k"
  Selector1/1 -> Demux/1  "y"
  one/1 -> Sum1/2, Sum2/2
  Sum1/1 -> Mux/2
  Sum2/1 -> Sum1/1, Mux/1
  Mux/1 -> Selector1/2

== system FKtest/Wave loads for heading1/Wave component loop/Force RAO tables/RAO interpolation in frequency6 ==
  Table : Inport
  omega : Inport  Port=2
  beta_idx : Inport  Port=3
  U_idx : Inport  Port=4
  Demux : Demux  Outputs=2
  Mux : Mux  Inputs=2
  Prelookup1 : PreLookup  BreakpointsData=vessel.forceRAO.w  BeginIndexSearchUsingPreviousIndexResult=on  ProcessOutOfRangeInput=Linear extrapolation
  Product : Product  RndMeth=Zero
  Selector1 : Selector  NumberOfDimensions=3  IndexOptions=Index vector (port),Index vector (port),Index vector (port)  Indices=[1 3],1,1  OutputSizes=1,1,1
  Sum1 : Sum  Inputs=++|
  Sum2 : Sum  Inputs=++|
  Sum3 : Sum  Inputs=-+|
  Sum4 : Sum  Inputs=++|
  one : Constant
  y : Outport
  wires:
  Prelookup1/1 -> Sum2/1
  Table/1 -> Selector1/1
  beta_idx/1 -> Selector1/3
  omega/1 -> Prelookup1/1
  U_idx/1 -> Selector1/4
  Sum4/1 -> y/1
  Sum3/1 -> Product/1
  Product/1 -> Sum4/2
  Demux/1 -> Sum4/1, Sum3/1  "y1"
  Demux/2 -> Sum3/2  "y2"
  Prelookup1/2 -> Product/2  "k"
  Selector1/1 -> Demux/1  "y"
  one/1 -> Sum1/2, Sum2/2
  Sum1/1 -> Mux/2
  Sum2/1 -> Sum1/1, Mux/1
  Mux/1 -> Selector1/2

== system FKtest/Wave loads for heading1/Wave component loop/Force RAO tables/RAO interpolation in frequency7 ==
  Table : Inport
  omega : Inport  Port=2
  beta_idx : Inport  Port=3
  U_idx : Inport  Port=4
  Demux : Demux  Outputs=2
  Mux : Mux  Inputs=2
  Prelookup1 : PreLookup  BreakpointsData=vessel.forceRAO.w  BeginIndexSearchUsingPreviousIndexResult=on  ProcessOutOfRangeInput=Linear extrapolation
  Product : Product  RndMeth=Zero
  Selector1 : Selector  NumberOfDimensions=3  IndexOptions=Index vector (port),Index vector (port),Index vector (port)  Indices=[1 3],1,1  OutputSizes=1,1,1
  Sum1 : Sum  Inputs=++|
  Sum2 : Sum  Inputs=++|
  Sum3 : Sum  Inputs=-+|
  Sum4 : Sum  Inputs=++|
  one : Constant
  y : Outport
  wires:
  Prelookup1/1 -> Sum2/1
  Table/1 -> Selector1/1
  beta_idx/1 -> Selector1/3
  omega/1 -> Prelookup1/1
  U_idx/1 -> Selector1/4
  Sum4/1 -> y/1
  Sum3/1 -> Product/1
  Product/1 -> Sum4/2
  Demux/1 -> Sum4/1, Sum3/1  "y1"
  Demux/2 -> Sum3/2  "y2"
  Prelookup1/2 -> Product/2  "k"
  Selector1/1 -> Demux/1  "y"
  one/1 -> Sum1/2, Sum2/2
  Sum1/1 -> Mux/2
  Sum2/1 -> Sum1/1, Mux/1
  Mux/1 -> Selector1/2

== system FKtest/Wave loads for heading1/Wave component loop/Force RAO tables/RAO interpolation in frequency8 ==
  Table : Inport
  omega : Inport  Port=2
  beta_idx : Inport  Port=3
  U_idx : Inport  Port=4
  Demux : Demux  Outputs=2
  Mux : Mux  Inputs=2
  Prelookup1 : PreLookup  BreakpointsData=vessel.forceRAO.w  BeginIndexSearchUsingPreviousIndexResult=on  ProcessOutOfRangeInput=Linear extrapolation
  Product : Product  RndMeth=Zero
  Selector1 : Selector  NumberOfDimensions=3  IndexOptions=Index vector (port),Index vector (port),Index vector (port)  Indices=[1 3],1,1  OutputSizes=1,1,1
  Sum1 : Sum  Inputs=++|
  Sum2 : Sum  Inputs=++|
  Sum3 : Sum  Inputs=-+|
  Sum4 : Sum  Inputs=++|
  one : Constant
  y : Outport
  wires:
  Prelookup1/1 -> Sum2/1
  Table/1 -> Selector1/1
  beta_idx/1 -> Selector1/3
  omega/1 -> Prelookup1/1
  U_idx/1 -> Selector1/4
  Sum4/1 -> y/1
  Sum3/1 -> Product/1
  Product/1 -> Sum4/2
  Demux/1 -> Sum4/1, Sum3/1  "y1"
  Demux/2 -> Sum3/2  "y2"
  Prelookup1/2 -> Product/2  "k"
  Selector1/1 -> Demux/1  "y"
  one/1 -> Sum1/2, Sum2/2
  Sum1/1 -> Mux/2
  Sum2/1 -> Sum1/1, Mux/1
  Mux/1 -> Selector1/2

== system FKtest/Wave loads for heading1/Wave component loop/Force RAO tables/RAO interpolation in frequency9 ==
  Table : Inport
  omega : Inport  Port=2
  beta_idx : Inport  Port=3
  U_idx : Inport  Port=4
  Demux : Demux  Outputs=2
  Mux : Mux  Inputs=2
  Prelookup1 : PreLookup  BreakpointsData=vessel.forceRAO.w  BeginIndexSearchUsingPreviousIndexResult=on  ProcessOutOfRangeInput=Linear extrapolation
  Product : Product  RndMeth=Zero
  Selector1 : Selector  NumberOfDimensions=3  IndexOptions=Index vector (port),Index vector (port),Index vector (port)  Indices=[1 3],1,1  OutputSizes=1,1,1
  Sum1 : Sum  Inputs=++|
  Sum2 : Sum  Inputs=++|
  Sum3 : Sum  Inputs=-+|
  Sum4 : Sum  Inputs=++|
  one : Constant
  y : Outport
  wires:
  Prelookup1/1 -> Sum2/1
  Table/1 -> Selector1/1
  beta_idx/1 -> Selector1/3
  omega/1 -> Prelookup1/1
  U_idx/1 -> Selector1/4
  Sum4/1 -> y/1
  Sum3/1 -> Product/1
  Product/1 -> Sum4/2
  Demux/1 -> Sum4/1, Sum3/1  "y1"
  Demux/2 -> Sum3/2  "y2"
  Prelookup1/2 -> Product/2  "k"
  Selector1/1 -> Demux/1  "y"
  one/1 -> Sum1/2, Sum2/2
  Sum1/1 -> Mux/2
  Sum2/1 -> Sum1/1, Mux/1
  Mux/1 -> Selector1/2

== system FKtest/Wave loads for heading1/Wave component loop/WD RAO tables/RAO interpolation in frequency1 ==
  Table : Inport
  omega : Inport  Port=2
  beta_idx : Inport  Port=3
  U_idx : Inport  Port=4
  Demux : Demux  Outputs=2
  Mux : Mux  Inputs=2
  Prelookup1 : PreLookup  BreakpointsData=vessel.forceRAO.w  BeginIndexSearchUsingPreviousIndexResult=on  ProcessOutOfRangeInput=Linear extrapolation
  Product : Product  RndMeth=Zero
  Selector1 : Selector  NumberOfDimensions=3  IndexOptions=Index vector (port),Index vector (port),Index vector (port)  Indices=[1 3],1,1  OutputSizes=1,1,1
  Sum1 : Sum  Inputs=++|
  Sum2 : Sum  Inputs=++|
  Sum3 : Sum  Inputs=-+|
  Sum4 : Sum  Inputs=++|
  one : Constant
  y : Outport
  wires:
  Prelookup1/1 -> Sum2/1
  Table/1 -> Selector1/1
  beta_idx/1 -> Selector1/3
  omega/1 -> Prelookup1/1
  U_idx/1 -> Selector1/4
  Sum4/1 -> y/1
  Sum3/1 -> Product/1
  Product/1 -> Sum4/2
  Demux/1 -> Sum4/1, Sum3/1  "y1"
  Demux/2 -> Sum3/2  "y2"
  Prelookup1/2 -> Product/2  "k"
  Selector1/1 -> Demux/1  "y"
  one/1 -> Sum1/2, Sum2/2
  Sum1/1 -> Mux/2
  Sum2/1 -> Sum1/1, Mux/1
  Mux/1 -> Selector1/2

== system FKtest/Wave loads for heading1/Wave component loop/WD RAO tables/RAO interpolation in frequency2 ==
  Table : Inport
  omega : Inport  Port=2
  beta_idx : Inport  Port=3
  U_idx : Inport  Port=4
  Demux : Demux  Outputs=2
  Mux : Mux  Inputs=2
  Prelookup1 : PreLookup  BreakpointsData=vessel.forceRAO.w  BeginIndexSearchUsingPreviousIndexResult=on  ProcessOutOfRangeInput=Linear extrapolation
  Product : Product  RndMeth=Zero
  Selector1 : Selector  NumberOfDimensions=3  IndexOptions=Index vector (port),Index vector (port),Index vector (port)  Indices=[1 3],1,1  OutputSizes=1,1,1
  Sum1 : Sum  Inputs=++|
  Sum2 : Sum  Inputs=++|
  Sum3 : Sum  Inputs=-+|
  Sum4 : Sum  Inputs=++|
  one : Constant
  y : Outport
  wires:
  Prelookup1/1 -> Sum2/1
  Table/1 -> Selector1/1
  beta_idx/1 -> Selector1/3
  omega/1 -> Prelookup1/1
  U_idx/1 -> Selector1/4
  Sum4/1 -> y/1
  Sum3/1 -> Product/1
  Product/1 -> Sum4/2
  Demux/1 -> Sum4/1, Sum3/1  "y1"
  Demux/2 -> Sum3/2  "y2"
  Prelookup1/2 -> Product/2  "k"
  Selector1/1 -> Demux/1  "y"
  one/1 -> Sum1/2, Sum2/2
  Sum1/1 -> Mux/2
  Sum2/1 -> Sum1/1, Mux/1
  Mux/1 -> Selector1/2

== system FKtest/Wave loads for heading1/Wave component loop/WD RAO tables/RAO interpolation in frequency3 ==
  Table : Inport
  omega : Inport  Port=2
  beta_idx : Inport  Port=3
  U_idx : Inport  Port=4
  Demux : Demux  Outputs=2
  Mux : Mux  Inputs=2
  Prelookup1 : PreLookup  BreakpointsData=vessel.forceRAO.w  BeginIndexSearchUsingPreviousIndexResult=on  ProcessOutOfRangeInput=Linear extrapolation
  Product : Product  RndMeth=Zero
  Selector1 : Selector  NumberOfDimensions=3  IndexOptions=Index vector (port),Index vector (port),Index vector (port)  Indices=[1 3],1,1  OutputSizes=1,1,1
  Sum1 : Sum  Inputs=++|
  Sum2 : Sum  Inputs=++|
  Sum3 : Sum  Inputs=-+|
  Sum4 : Sum  Inputs=++|
  one : Constant
  y : Outport
  wires:
  Prelookup1/1 -> Sum2/1
  Table/1 -> Selector1/1
  beta_idx/1 -> Selector1/3
  omega/1 -> Prelookup1/1
  U_idx/1 -> Selector1/4
  Sum4/1 -> y/1
  Sum3/1 -> Product/1
  Product/1 -> Sum4/2
  Demux/1 -> Sum4/1, Sum3/1  "y1"
  Demux/2 -> Sum3/2  "y2"
  Prelookup1/2 -> Product/2  "k"
  Selector1/1 -> Demux/1  "y"
  one/1 -> Sum1/2, Sum2/2
  Sum1/1 -> Mux/2
  Sum2/1 -> Sum1/1, Mux/1
  Mux/1 -> Selector1/2

== system FKtest/Wave loads for heading2/Wave component loop/Force RAO tables/RAO interpolation in frequency1 ==
  Table : Inport
  omega : Inport  Port=2
  beta_idx : Inport  Port=3
  U_idx : Inport  Port=4
  Demux : Demux  Outputs=2
  Mux : Mux  Inputs=2
  Prelookup1 : PreLookup  BreakpointsData=vessel.forceRAO.w  BeginIndexSearchUsingPreviousIndexResult=on  ProcessOutOfRangeInput=Linear extrapolation
  Product : Product  RndMeth=Zero
  Selector1 : Selector  NumberOfDimensions=3  IndexOptions=Index vector (port),Index vector (port),Index vector (port)  Indices=[1 3],1,1  OutputSizes=1,1,1
  Sum1 : Sum  Inputs=++|
  Sum2 : Sum  Inputs=++|
  Sum3 : Sum  Inputs=-+|
  Sum4 : Sum  Inputs=++|
  one : Constant
  y : Outport
  wires:
  Prelookup1/1 -> Sum2/1
  Table/1 -> Selector1/1
  beta_idx/1 -> Selector1/3
  omega/1 -> Prelookup1/1
  U_idx/1 -> Selector1/4
  Sum4/1 -> y/1
  Sum3/1 -> Product/1
  Product/1 -> Sum4/2
  Demux/1 -> Sum4/1, Sum3/1  "y1"
  Demux/2 -> Sum3/2  "y2"
  Prelookup1/2 -> Product/2  "k"
  Selector1/1 -> Demux/1  "y"
  one/1 -> Sum1/2, Sum2/2
  Sum1/1 -> Mux/2
  Sum2/1 -> Sum1/1, Mux/1
  Mux/1 -> Selector1/2

== system FKtest/Wave loads for heading2/Wave component loop/Force RAO tables/RAO interpolation in frequency10 ==
  Table : Inport
  omega : Inport  Port=2
  beta_idx : Inport  Port=3
  U_idx : Inport  Port=4
  Demux : Demux  Outputs=2
  Mux : Mux  Inputs=2
  Prelookup1 : PreLookup  BreakpointsData=vessel.forceRAO.w  BeginIndexSearchUsingPreviousIndexResult=on  ProcessOutOfRangeInput=Linear extrapolation
  Product : Product  RndMeth=Zero
  Selector1 : Selector  NumberOfDimensions=3  IndexOptions=Index vector (port),Index vector (port),Index vector (port)  Indices=[1 3],1,1  OutputSizes=1,1,1
  Sum1 : Sum  Inputs=++|
  Sum2 : Sum  Inputs=++|
  Sum3 : Sum  Inputs=-+|
  Sum4 : Sum  Inputs=++|
  one : Constant
  y : Outport
  wires:
  Prelookup1/1 -> Sum2/1
  Table/1 -> Selector1/1
  beta_idx/1 -> Selector1/3
  omega/1 -> Prelookup1/1
  U_idx/1 -> Selector1/4
  Sum4/1 -> y/1
  Sum3/1 -> Product/1
  Product/1 -> Sum4/2
  Demux/1 -> Sum4/1, Sum3/1  "y1"
  Demux/2 -> Sum3/2  "y2"
  Prelookup1/2 -> Product/2  "k"
  Selector1/1 -> Demux/1  "y"
  one/1 -> Sum1/2, Sum2/2
  Sum1/1 -> Mux/2
  Sum2/1 -> Sum1/1, Mux/1
  Mux/1 -> Selector1/2

== system FKtest/Wave loads for heading2/Wave component loop/Force RAO tables/RAO interpolation in frequency11 ==
  Table : Inport
  omega : Inport  Port=2
  beta_idx : Inport  Port=3
  U_idx : Inport  Port=4
  Demux : Demux  Outputs=2
  Mux : Mux  Inputs=2
  Prelookup1 : PreLookup  BreakpointsData=vessel.forceRAO.w  BeginIndexSearchUsingPreviousIndexResult=on  ProcessOutOfRangeInput=Linear extrapolation
  Product : Product  RndMeth=Zero
  Selector1 : Selector  NumberOfDimensions=3  IndexOptions=Index vector (port),Index vector (port),Index vector (port)  Indices=[1 3],1,1  OutputSizes=1,1,1
  Sum1 : Sum  Inputs=++|
  Sum2 : Sum  Inputs=++|
  Sum3 : Sum  Inputs=-+|
  Sum4 : Sum  Inputs=++|
  one : Constant
  y : Outport
  wires:
  Prelookup1/1 -> Sum2/1
  Table/1 -> Selector1/1
  beta_idx/1 -> Selector1/3
  omega/1 -> Prelookup1/1
  U_idx/1 -> Selector1/4
  Sum4/1 -> y/1
  Sum3/1 -> Product/1
  Product/1 -> Sum4/2
  Demux/1 -> Sum4/1, Sum3/1  "y1"
  Demux/2 -> Sum3/2  "y2"
  Prelookup1/2 -> Product/2  "k"
  Selector1/1 -> Demux/1  "y"
  one/1 -> Sum1/2, Sum2/2
  Sum1/1 -> Mux/2
  Sum2/1 -> Sum1/1, Mux/1
  Mux/1 -> Selector1/2

== system FKtest/Wave loads for heading2/Wave component loop/Force RAO tables/RAO interpolation in frequency12 ==
  Table : Inport
  omega : Inport  Port=2
  beta_idx : Inport  Port=3
  U_idx : Inport  Port=4
  Demux : Demux  Outputs=2
  Mux : Mux  Inputs=2
  Prelookup1 : PreLookup  BreakpointsData=vessel.forceRAO.w  BeginIndexSearchUsingPreviousIndexResult=on  ProcessOutOfRangeInput=Linear extrapolation
  Product : Product  RndMeth=Zero
  Selector1 : Selector  NumberOfDimensions=3  IndexOptions=Index vector (port),Index vector (port),Index vector (port)  Indices=[1 3],1,1  OutputSizes=1,1,1
  Sum1 : Sum  Inputs=++|
  Sum2 : Sum  Inputs=++|
  Sum3 : Sum  Inputs=-+|
  Sum4 : Sum  Inputs=++|
  one : Constant
  y : Outport
  wires:
  Prelookup1/1 -> Sum2/1
  Table/1 -> Selector1/1
  beta_idx/1 -> Selector1/3
  omega/1 -> Prelookup1/1
  U_idx/1 -> Selector1/4
  Sum4/1 -> y/1
  Sum3/1 -> Product/1
  Product/1 -> Sum4/2
  Demux/1 -> Sum4/1, Sum3/1  "y1"
  Demux/2 -> Sum3/2  "y2"
  Prelookup1/2 -> Product/2  "k"
  Selector1/1 -> Demux/1  "y"
  one/1 -> Sum1/2, Sum2/2
  Sum1/1 -> Mux/2
  Sum2/1 -> Sum1/1, Mux/1
  Mux/1 -> Selector1/2

== system FKtest/Wave loads for heading2/Wave component loop/Force RAO tables/RAO interpolation in frequency2 ==
  Table : Inport
  omega : Inport  Port=2
  beta_idx : Inport  Port=3
  U_idx : Inport  Port=4
  Demux : Demux  Outputs=2
  Mux : Mux  Inputs=2
  Prelookup1 : PreLookup  BreakpointsData=vessel.forceRAO.w  BeginIndexSearchUsingPreviousIndexResult=on  ProcessOutOfRangeInput=Linear extrapolation
  Product : Product  RndMeth=Zero
  Selector1 : Selector  NumberOfDimensions=3  IndexOptions=Index vector (port),Index vector (port),Index vector (port)  Indices=[1 3],1,1  OutputSizes=1,1,1
  Sum1 : Sum  Inputs=++|
  Sum2 : Sum  Inputs=++|
  Sum3 : Sum  Inputs=-+|
  Sum4 : Sum  Inputs=++|
  one : Constant
  y : Outport
  wires:
  Prelookup1/1 -> Sum2/1
  Table/1 -> Selector1/1
  beta_idx/1 -> Selector1/3
  omega/1 -> Prelookup1/1
  U_idx/1 -> Selector1/4
  Sum4/1 -> y/1
  Sum3/1 -> Product/1
  Product/1 -> Sum4/2
  Demux/1 -> Sum4/1, Sum3/1  "y1"
  Demux/2 -> Sum3/2  "y2"
  Prelookup1/2 -> Product/2  "k"
  Selector1/1 -> Demux/1  "y"
  one/1 -> Sum1/2, Sum2/2
  Sum1/1 -> Mux/2
  Sum2/1 -> Sum1/1, Mux/1
  Mux/1 -> Selector1/2

== system FKtest/Wave loads for heading2/Wave component loop/Force RAO tables/RAO interpolation in frequency3 ==
  Table : Inport
  omega : Inport  Port=2
  beta_idx : Inport  Port=3
  U_idx : Inport  Port=4
  Demux : Demux  Outputs=2
  Mux : Mux  Inputs=2
  Prelookup1 : PreLookup  BreakpointsData=vessel.forceRAO.w  BeginIndexSearchUsingPreviousIndexResult=on  ProcessOutOfRangeInput=Linear extrapolation
  Product : Product  RndMeth=Zero
  Selector1 : Selector  NumberOfDimensions=3  IndexOptions=Index vector (port),Index vector (port),Index vector (port)  Indices=[1 3],1,1  OutputSizes=1,1,1
  Sum1 : Sum  Inputs=++|
  Sum2 : Sum  Inputs=++|
  Sum3 : Sum  Inputs=-+|
  Sum4 : Sum  Inputs=++|
  one : Constant
  y : Outport
  wires:
  Prelookup1/1 -> Sum2/1
  Table/1 -> Selector1/1
  beta_idx/1 -> Selector1/3
  omega/1 -> Prelookup1/1
  U_idx/1 -> Selector1/4
  Sum4/1 -> y/1
  Sum3/1 -> Product/1
  Product/1 -> Sum4/2
  Demux/1 -> Sum4/1, Sum3/1  "y1"
  Demux/2 -> Sum3/2  "y2"
  Prelookup1/2 -> Product/2  "k"
  Selector1/1 -> Demux/1  "y"
  one/1 -> Sum1/2, Sum2/2
  Sum1/1 -> Mux/2
  Sum2/1 -> Sum1/1, Mux/1
  Mux/1 -> Selector1/2

== system FKtest/Wave loads for heading2/Wave component loop/Force RAO tables/RAO interpolation in frequency4 ==
  Table : Inport
  omega : Inport  Port=2
  beta_idx : Inport  Port=3
  U_idx : Inport  Port=4
  Demux : Demux  Outputs=2
  Mux : Mux  Inputs=2
  Prelookup1 : PreLookup  BreakpointsData=vessel.forceRAO.w  BeginIndexSearchUsingPreviousIndexResult=on  ProcessOutOfRangeInput=Linear extrapolation
  Product : Product  RndMeth=Zero
  Selector1 : Selector  NumberOfDimensions=3  IndexOptions=Index vector (port),Index vector (port),Index vector (port)  Indices=[1 3],1,1  OutputSizes=1,1,1
  Sum1 : Sum  Inputs=++|
  Sum2 : Sum  Inputs=++|
  Sum3 : Sum  Inputs=-+|
  Sum4 : Sum  Inputs=++|
  one : Constant
  y : Outport
  wires:
  Prelookup1/1 -> Sum2/1
  Table/1 -> Selector1/1
  beta_idx/1 -> Selector1/3
  omega/1 -> Prelookup1/1
  U_idx/1 -> Selector1/4
  Sum4/1 -> y/1
  Sum3/1 -> Product/1
  Product/1 -> Sum4/2
  Demux/1 -> Sum4/1, Sum3/1  "y1"
  Demux/2 -> Sum3/2  "y2"
  Prelookup1/2 -> Product/2  "k"
  Selector1/1 -> Demux/1  "y"
  one/1 -> Sum1/2, Sum2/2
  Sum1/1 -> Mux/2
  Sum2/1 -> Sum1/1, Mux/1
  Mux/1 -> Selector1/2
